simulink model "lab1simu"  (Simulink 7.7)
settings: Solver=ode45  StartTime=0.0  StopTime=1000  RelTol=1e-3
settings Model: Creator=student  LastModifiedBy=mestan

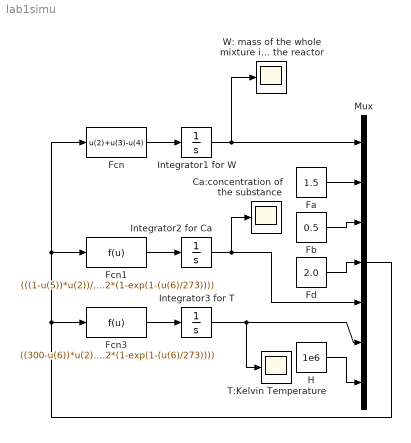
== system lab1simu ==
  " Ca:concentration of the substance" : Scope
  Fa : Constant  Value=1.5
  Fb : Constant  Value=0.5
  Fcn : Fcn  Expr=u(2)+u(3)-u(4)
  Fcn1 : Fcn  Expr=(((1-u(5))*u(2))/u(1))-(u(5)*u(3)/u(1))-(u(5)*0.2*(1-exp(1-(u(6)/273))))
  Fcn3 : Fcn  Expr=((300-u(6))*u(2)/u(1)) + ((300-u(6))*u(3)/u(1)) + (u(7)/(5000*u(1))) - (0.1*u(5)*0.2*(1-exp(1-(u(6)/273))))
  Fd : Constant  Value=2.0
  H : Constant  Value=1e6
  Integrator1 for W : Integrator  InitialCondition=500
  Integrator2 for Ca : Integrator  InitialCondition=1
  Integrator3 for T : Integrator  InitialCondition=300
  Mux : Mux  Inputs=7
  T:Kelvin Temperature : Scope
      settings: TimeRange=100  SaveName=ScopeData2
  W: mass of the whole mixture in the reactor : Scope
  wires:
  Integrator1 for W/1 -> Mux/1, W: mass of the whole mixture in the reactor/1
  Fa/1 -> Mux/2
  Fb/1 -> Mux/3
  Fd/1 -> Mux/4
  Mux/1 -> Fcn3/1, Fcn/1, Fcn1/1
  Fcn/1 -> Integrator1 for W/1
  Fcn1/1 -> Integrator2 for Ca/1
  Fcn3/1 -> Integrator3 for T/1
  Integrator2 for Ca/1 -> Mux/5, " Ca:concentration of the substance"/1
  Integrator3 for T/1 -> Mux/6, T:Kelvin Temperature/1
  H/1 -> Mux/7
